simulink library "TURING_LOGIC"  (R2019b)
settings: Solver=VariableStepAuto  StartTime=0.0  StopTime=10.0  RelTol=1e-3
libraries: $bdroot x162, NOT x29, NAND x4
settings Model: Creator=jthur  LastModifiedBy=JTHURT

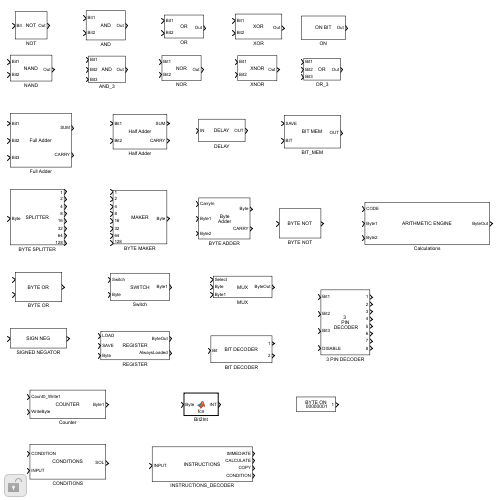
[thumbnail: Simulink's stored preview of the top-level diagram]
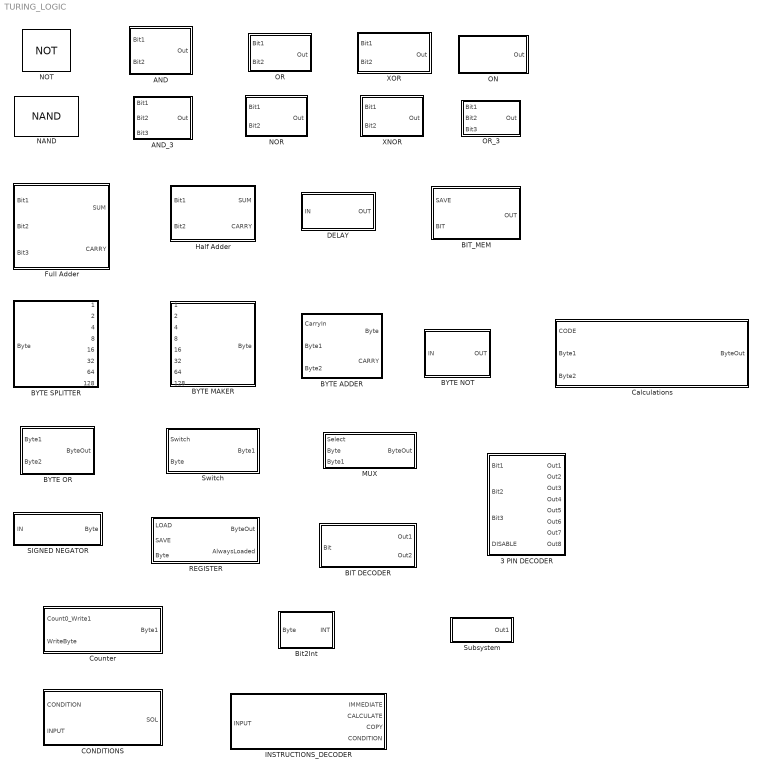
== system TURING_LOGIC ==
  3 PIN DECODER : Subsystem
      mask Display: fprintf("3 \n PIN \n DECODER")
  AND : Subsystem
      mask Display: fprintf("AND")
  AND_3 : Subsystem
      mask Display: fprintf("AND")
  BIT DECODER : Subsystem
      mask Display: fprintf("BIT DECODER")
  BIT_MEM : Subsystem
      mask Display: fprintf("BIT MEM")
  BYTE ADDER : Subsystem
      mask Display: fprintf("  Byte \n Adder")
  BYTE MAKER : Subsystem
      mask Display: fprintf("MAKER")
  BYTE NOT : Subsystem
      mask Display: fprintf("BYTE NOT")
  BYTE OR : Subsystem
      mask Display: fprintf("BYTE OR")
  "BYTE SPLITTER " : Subsystem
      mask Display: fprintf("SPLITTER")
  Bit2Int : MATLAB Function  TreatAsAtomicUnit=on
  CONDITIONS : Subsystem
      mask Display: fprintf("CONDITIONS")
  Calculations : Subsystem
      mask Display: fprintf("ARITHMETIC ENGINE")
  Counter : Subsystem
      mask Display: fprintf("COUNTER")
  DELAY : Subsystem
      mask Display: fprintf("DELAY")
  Full Adder : Subsystem
      mask Display: fprintf("Full Adder")
  Half Adder : Subsystem
      mask Display: fprintf("Half Adder")
  INSTRUCTIONS_DECODER : Subsystem
      mask Display: fprintf("INSTRUCTIONS")
  MUX : Subsystem
      mask Display: fprintf("MUX")
  NAND : NAND/NAND  SystemSampleTime=-1  Latency=0  AutoFrameSizeCalculation=off
  NOR : Subsystem
      mask Display: fprintf("NOR")
  NOT : NOT/NOT  SystemSampleTime=-1  Latency=0  AutoFrameSizeCalculation=off
  ON : Subsystem
      mask Display: fprintf("ON BIT")
  OR : Subsystem
      mask Display: fprintf("OR")
  OR_3 : Subsystem
      mask Display: fprintf("OR")
  REGISTER : Subsystem
      mask Display: fprintf("REGISTER")
  SIGNED NEGATOR : Subsystem
      mask Display: fprintf("SIGN NEG")
  Subsystem : Subsystem
      mask Display: fprintf("BYTE ON\n 00000001")
  Switch : Subsystem
      mask Display: fprintf("SWITCH")
  XNOR : Subsystem
      mask Display: fprintf("XNOR")
  XOR : Subsystem
      mask Display: fprintf("XOR")

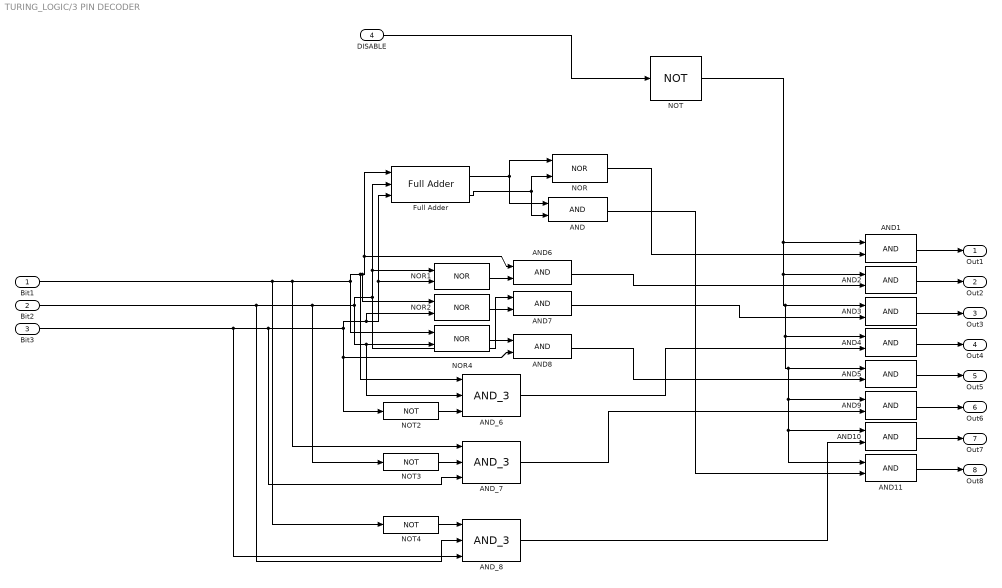
== system TURING_LOGIC/3 PIN DECODER ==
  Bit1 : Inport
  Bit2 : Inport  Port=2
  Bit3 : Inport  Port=3
  DISABLE : Inport  Port=4
  AND{,1..11} (12 alike) : $bdroot/AND  SystemSampleTime=-1  Latency=0  AutoFrameSizeCalculation=off
  AND_6 : $bdroot/AND_3  SystemSampleTime=-1  Latency=0  AutoFrameSizeCalculation=off
  AND_7 : $bdroot/AND_3  SystemSampleTime=-1  Latency=0  AutoFrameSizeCalculation=off
  AND_8 : $bdroot/AND_3  SystemSampleTime=-1  Latency=0  AutoFrameSizeCalculation=off
  Full Adder : $bdroot/Full Adder  SystemSampleTime=-1  Latency=0  AutoFrameSizeCalculation=off
  NOR{,1..2,4} (4 alike) : $bdroot/NOR  SystemSampleTime=-1  Latency=0  AutoFrameSizeCalculation=off
  NOT{,2..4} (4 alike) : NOT/NOT  SystemSampleTime=-1  Latency=0  AutoFrameSizeCalculation=off
  Out1 : Outport
  Out2 : Outport  Port=2
  Out3 : Outport  Port=3
  Out4 : Outport  Port=4
  Out5 : Outport  Port=5
  Out6 : Outport  Port=6
  Out7 : Outport  Port=7
  Out8 : Outport  Port=8
  wires:
  Bit3/1 -> AND_8/3, AND_7/3, NOR2/2, Full Adder/3, NOR1/2, NOT2/1, AND8/2
  Full Adder/2 -> NOR/2, AND/2
  Bit2/1 -> AND_8/2, NOT3/1, Full Adder/2, NOR1/1, AND7/1, AND_6/2, NOR4/2
  Bit1/1 -> NOT4/1, AND_7/1, AND_6/1, NOR2/1, Full Adder/1, AND6/1, NOR4/1
  NOT2/1 -> AND_6/3
  NOT3/1 -> AND_7/2
  NOR2/1 -> AND7/2
  NOR4/1 -> AND8/1
  NOR1/1 -> AND6/2
  NOT4/1 -> AND_8/1
  Full Adder/1 -> AND/1, NOR/1
  AND1/1 -> Out1/1
  AND2/1 -> Out2/1
  AND3/1 -> Out3/1
  AND4/1 -> Out4/1
  AND5/1 -> Out5/1
  AND9/1 -> Out6/1
  AND10/1 -> Out7/1
  AND11/1 -> Out8/1
  NOT/1 -> AND11/1, AND10/1, AND9/1, AND5/1, AND4/1, AND3/1, AND2/1, AND1/1
  AND/1 -> AND11/2
  NOR/1 -> AND1/2
  AND6/1 -> AND2/2
  AND7/1 -> AND3/2
  AND8/1 -> AND5/2
  AND_6/1 -> AND4/2
  AND_7/1 -> AND9/2
  AND_8/1 -> AND10/2
  DISABLE/1 -> NOT/1

== system TURING_LOGIC/AND ==
  Bit1 : Inport
  Bit2 : Inport  Port=2
  NAND1 : NAND/NAND  SystemSampleTime=-1  Latency=0  AutoFrameSizeCalculation=off
  NOT1 : NOT/NOT  SystemSampleTime=-1  Latency=0  AutoFrameSizeCalculation=off
  Out : Outport
  wires:
  NAND1/1 -> NOT1/1
  Bit1/1 -> NAND1/1
  NOT1/1 -> Out/1
  Bit2/1 -> NAND1/2

== system TURING_LOGIC/AND_3 ==
  Bit1 : Inport
  Bit2 : Inport  Port=2
  Bit3 : Inport  Port=3
  AND1 : $bdroot/AND  SystemSampleTime=-1  Latency=0  AutoFrameSizeCalculation=off
  AND2 : $bdroot/AND  SystemSampleTime=-1  Latency=0  AutoFrameSizeCalculation=off
  Out : Outport
  wires:
  AND1/1 -> AND2/1
  AND2/1 -> Out/1
  Bit1/1 -> AND1/1
  Bit3/1 -> AND2/2
  Bit2/1 -> AND1/2

== system TURING_LOGIC/BIT DECODER ==
  Bit : Inport
  AND : $bdroot/AND  SystemSampleTime=-1  Latency=0  AutoFrameSizeCalculation=off
  AND1 : $bdroot/AND  SystemSampleTime=-1  Latency=0  AutoFrameSizeCalculation=off
  NOT : NOT/NOT  SystemSampleTime=-1  Latency=0  AutoFrameSizeCalculation=off
  ON : $bdroot/ON  SystemSampleTime=-1  Latency=0  AutoFrameSizeCalculation=off
  Out1 : Outport
  Out2 : Outport  Port=2
  wires:
  ON/1 -> AND/2, AND1/2
  Bit/1 -> AND1/1, NOT/1
  NOT/1 -> AND/1
  AND/1 -> Out1/1
  AND1/1 -> Out2/1

== system TURING_LOGIC/BIT_MEM ==
  SAVE : Inport
  BIT : Inport  Port=2
  AND : $bdroot/AND  SystemSampleTime=-1  Latency=0  AutoFrameSizeCalculation=off
  AND1 : $bdroot/AND  SystemSampleTime=-1  Latency=0  AutoFrameSizeCalculation=off
  DELAY : $bdroot/DELAY  SystemSampleTime=-1  Latency=0  AutoFrameSizeCalculation=off
  NOR : $bdroot/NOR  SystemSampleTime=-1  Latency=0  AutoFrameSizeCalculation=off
  NOR1 : $bdroot/NOR  SystemSampleTime=-1  Latency=0  AutoFrameSizeCalculation=off
  NOT : NOT/NOT  SystemSampleTime=-1  Latency=0  AutoFrameSizeCalculation=off
  OUT : Outport
  wires:
  BIT/1 -> AND1/2, NOT/1
  NOT/1 -> AND/2
  SAVE/1 -> AND/1, AND1/1
  AND/1 -> NOR1/2
  NOR1/1 -> DELAY/1
  AND1/1 -> NOR/1
  NOR/1 -> NOR1/1
  DELAY/1 -> OUT/1, NOR/2

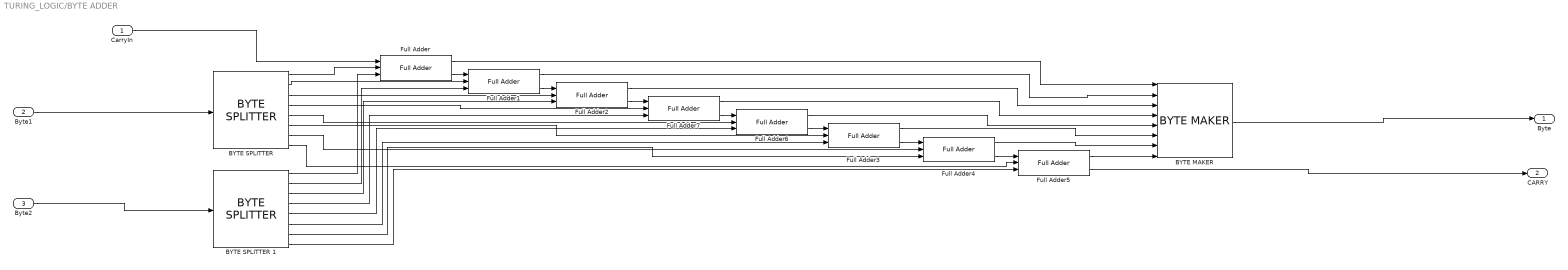
== system TURING_LOGIC/BYTE ADDER ==
  CarryIn : Inport
  Byte1 : Inport  Port=2
  Byte2 : Inport  Port=3
  BYTE MAKER : $bdroot/BYTE MAKER  SystemSampleTime=-1  Latency=0  AutoFrameSizeCalculation=off
  "BYTE SPLITTER " : $bdroot/BYTE SPLITTER   SystemSampleTime=-1  Latency=0  AutoFrameSizeCalculation=off
  BYTE SPLITTER 1 : $bdroot/BYTE SPLITTER   SystemSampleTime=-1  Latency=0  AutoFrameSizeCalculation=off
  Full Adder{,1..7} (8 alike) : $bdroot/Full Adder  SystemSampleTime=-1  Latency=0  AutoFrameSizeCalculation=off
  Byte : Outport
  CARRY : Outport  Port=2
  wires:
  BYTE SPLITTER 1/5 -> Full Adder6/3
  BYTE SPLITTER 1/3 -> Full Adder2/3
  "BYTE SPLITTER "/7 -> Full Adder4/2
  Full Adder1/1 -> BYTE MAKER/2
  BYTE SPLITTER 1/4 -> Full Adder7/3
  Full Adder3/2 -> Full Adder4/1
  "BYTE SPLITTER "/4 -> Full Adder7/2
  "BYTE SPLITTER "/5 -> Full Adder6/2
  Full Adder/1 -> BYTE MAKER/1
  Full Adder6/2 -> Full Adder3/1
  Full Adder3/1 -> BYTE MAKER/6
  Byte2/1 -> BYTE SPLITTER 1/1
  BYTE SPLITTER 1/6 -> Full Adder3/3
  BYTE SPLITTER 1/2 -> Full Adder1/3
  Full Adder/2 -> Full Adder1/1
  BYTE SPLITTER 1/8 -> Full Adder5/3
  Full Adder4/1 -> BYTE MAKER/7
  "BYTE SPLITTER "/2 -> Full Adder1/2
  Full Adder6/1 -> BYTE MAKER/5
  "BYTE SPLITTER "/1 -> Full Adder/2
  Full Adder2/1 -> BYTE MAKER/3
  Full Adder1/2 -> Full Adder2/1
  "BYTE SPLITTER "/3 -> Full Adder2/2
  Full Adder5/2 -> CARRY/1
  BYTE SPLITTER 1/1 -> Full Adder/3
  Full Adder7/1 -> BYTE MAKER/4
  "BYTE SPLITTER "/8 -> Full Adder5/2
  Full Adder5/1 -> BYTE MAKER/8
  "BYTE SPLITTER "/6 -> Full Adder3/2
  Full Adder2/2 -> Full Adder7/1
  BYTE SPLITTER 1/7 -> Full Adder4/3
  Full Adder7/2 -> Full Adder6/1
  CarryIn/1 -> Full Adder/1
  Full Adder4/2 -> Full Adder5/1
  BYTE MAKER/1 -> Byte/1
  Byte1/1 -> "BYTE SPLITTER "/1

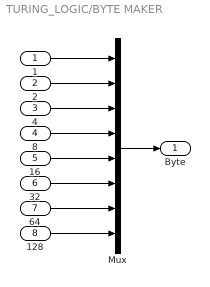
== system TURING_LOGIC/BYTE MAKER ==
  1 : Inport
  2 : Inport  Port=2
  4 : Inport  Port=3
  8 : Inport  Port=4
  16 : Inport  Port=5
  32 : Inport  Port=6
  64 : Inport  Port=7
  128 : Inport  Port=8
  Mux : Mux  Inputs=8
  Byte : Outport
  wires:
  1/1 -> Mux/1
  2/1 -> Mux/2
  4/1 -> Mux/3
  8/1 -> Mux/4
  16/1 -> Mux/5
  32/1 -> Mux/6
  64/1 -> Mux/7
  128/1 -> Mux/8
  Mux/1 -> Byte/1

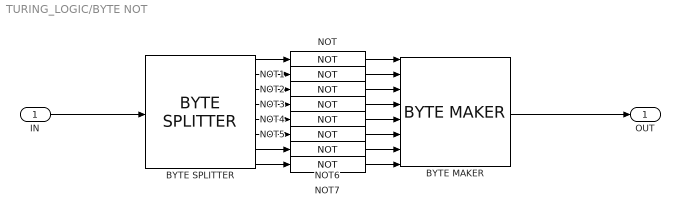
== system TURING_LOGIC/BYTE NOT ==
  IN : Inport
  BYTE MAKER : $bdroot/BYTE MAKER  SystemSampleTime=-1  Latency=0  AutoFrameSizeCalculation=off
  "BYTE SPLITTER " : $bdroot/BYTE SPLITTER   SystemSampleTime=-1  Latency=0  AutoFrameSizeCalculation=off
  NOT{,1..7} (8 alike) : NOT/NOT  SystemSampleTime=-1  Latency=0  AutoFrameSizeCalculation=off
  OUT : Outport
  wires:
  "BYTE SPLITTER "/8 -> NOT7/1
  NOT4/1 -> BYTE MAKER/5
  NOT/1 -> BYTE MAKER/1
  "BYTE SPLITTER "/3 -> NOT2/1
  "BYTE SPLITTER "/7 -> NOT6/1
  "BYTE SPLITTER "/4 -> NOT3/1
  NOT6/1 -> BYTE MAKER/7
  NOT7/1 -> BYTE MAKER/8
  "BYTE SPLITTER "/5 -> NOT4/1
  NOT2/1 -> BYTE MAKER/3
  NOT5/1 -> BYTE MAKER/6
  "BYTE SPLITTER "/2 -> NOT1/1
  NOT1/1 -> BYTE MAKER/2
  "BYTE SPLITTER "/1 -> NOT/1
  IN/1 -> "BYTE SPLITTER "/1
  NOT3/1 -> BYTE MAKER/4
  "BYTE SPLITTER "/6 -> NOT5/1
  BYTE MAKER/1 -> OUT/1

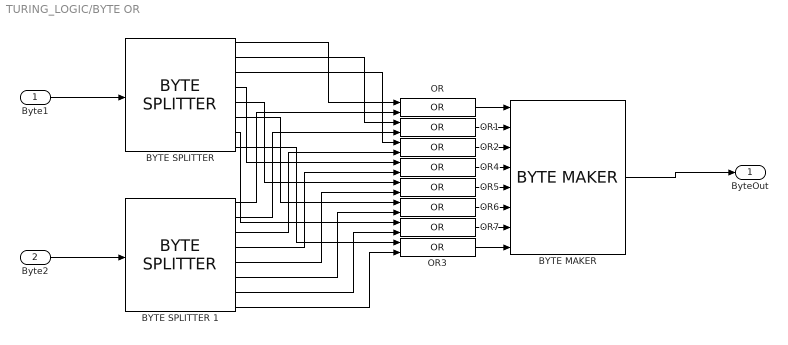
== system TURING_LOGIC/BYTE OR ==
  Byte1 : Inport
  Byte2 : Inport  Port=2
  BYTE MAKER : $bdroot/BYTE MAKER  SystemSampleTime=-1  Latency=0  AutoFrameSizeCalculation=off
  "BYTE SPLITTER " : $bdroot/BYTE SPLITTER   SystemSampleTime=-1  Latency=0  AutoFrameSizeCalculation=off
  BYTE SPLITTER 1 : $bdroot/BYTE SPLITTER   SystemSampleTime=-1  Latency=0  AutoFrameSizeCalculation=off
  OR{,1..7} (8 alike) : $bdroot/OR  SystemSampleTime=-1  Latency=0  AutoFrameSizeCalculation=off
  ByteOut : Outport
  wires:
  "BYTE SPLITTER "/2 -> OR1/1
  OR2/1 -> BYTE MAKER/3
  BYTE SPLITTER 1/2 -> OR1/2
  OR5/1 -> BYTE MAKER/5
  "BYTE SPLITTER "/3 -> OR2/1
  BYTE SPLITTER 1/1 -> OR/2
  BYTE SPLITTER 1/5 -> OR5/2
  BYTE SPLITTER 1/8 -> OR3/2
  BYTE SPLITTER 1/7 -> OR7/2
  "BYTE SPLITTER "/6 -> OR6/1
  OR3/1 -> BYTE MAKER/8
  BYTE SPLITTER 1/4 -> OR4/2
  BYTE SPLITTER 1/6 -> OR6/2
  BYTE SPLITTER 1/3 -> OR2/2
  Byte2/1 -> BYTE SPLITTER 1/1
  "BYTE SPLITTER "/4 -> OR4/1
  OR7/1 -> BYTE MAKER/7
  "BYTE SPLITTER "/5 -> OR5/1
  OR1/1 -> BYTE MAKER/2
  OR/1 -> BYTE MAKER/1
  OR4/1 -> BYTE MAKER/4
  "BYTE SPLITTER "/1 -> OR/1
  "BYTE SPLITTER "/8 -> OR3/1
  OR6/1 -> BYTE MAKER/6
  "BYTE SPLITTER "/7 -> OR7/1
  Byte1/1 -> "BYTE SPLITTER "/1
  BYTE MAKER/1 -> ByteOut/1

== system TURING_LOGIC/BYTE SPLITTER  ==
  Byte : Inport
  Demux : Demux  Outputs=8
  1 : Outport
  2 : Outport  Port=2
  4 : Outport  Port=3
  8 : Outport  Port=4
  16 : Outport  Port=5
  32 : Outport  Port=6
  64 : Outport  Port=7
  128 : Outport  Port=8
  wires:
  Byte/1 -> Demux/1
  Demux/1 -> 1/1
  Demux/2 -> 2/1
  Demux/3 -> 4/1
  Demux/4 -> 8/1
  Demux/5 -> 16/1
  Demux/6 -> 32/1
  Demux/7 -> 64/1
  Demux/8 -> 128/1

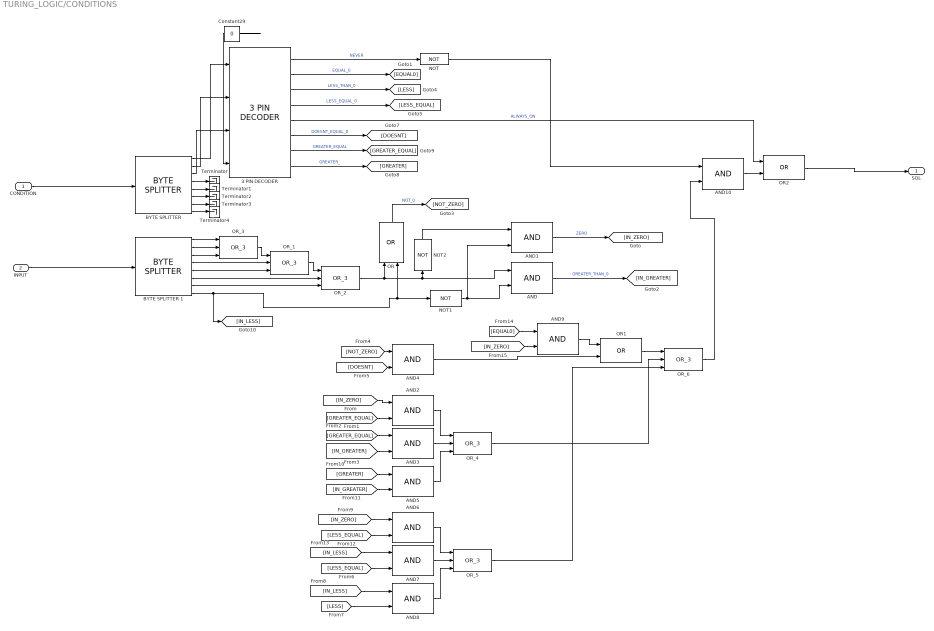
== system TURING_LOGIC/CONDITIONS ==
  CONDITION : Inport
  INPUT : Inport  Port=2
  3 PIN DECODER : $bdroot/3 PIN DECODER  SystemSampleTime=-1  Latency=0  AutoFrameSizeCalculation=off
  AND{,1..10} (11 alike) : $bdroot/AND  SystemSampleTime=-1  Latency=0  AutoFrameSizeCalculation=off
  "BYTE SPLITTER " : $bdroot/BYTE SPLITTER   SystemSampleTime=-1  Latency=0  AutoFrameSizeCalculation=off
  BYTE SPLITTER 1 : $bdroot/BYTE SPLITTER   SystemSampleTime=-1  Latency=0  AutoFrameSizeCalculation=off
  Constant29 : Constant  Value=0  SampleTime=-1
  NOT : NOT/NOT  SystemSampleTime=-1  Latency=0  AutoFrameSizeCalculation=off
  NOT1 : NOT/NOT  SystemSampleTime=-1  Latency=0  AutoFrameSizeCalculation=off
  NOT2 : NOT/NOT  SystemSampleTime=-1  Latency=0  AutoFrameSizeCalculation=off
  OR : $bdroot/OR  SystemSampleTime=-1  Latency=0  AutoFrameSizeCalculation=off
  OR1 : $bdroot/OR  SystemSampleTime=-1  Latency=0  AutoFrameSizeCalculation=off
  OR2 : $bdroot/OR  SystemSampleTime=-1  Latency=0  AutoFrameSizeCalculation=off
  OR_{1..6} (6 alike) : $bdroot/OR_3  SystemSampleTime=-1  Latency=0  AutoFrameSizeCalculation=off
  Terminator{,1..4} (5 alike) : Terminator
  SOL : Outport
  wires:
  [LESS_EQUAL] -> AND7/2
  BYTE SPLITTER 1/8 -> [IN_LESS], NOT1/1, OR/2
  BYTE SPLITTER 1/6 -> OR_2/2
  NOT1/1 -> AND1/2, AND/2
  [IN_ZERO] -> AND2/1
  BYTE SPLITTER 1/7 -> OR_2/3
  OR_6/1 -> AND10/2
  NOT2/1 -> AND1/1
  3 PIN DECODER/6 -> [DOESNT]  "DOESNT_EQUAL_0"
  OR_3/1 -> OR_1/1
  OR1/1 -> OR_6/1
  [IN_ZERO] -> AND6/1
  AND5/1 -> OR_4/3
  [IN_LESS] -> AND7/1
  "BYTE SPLITTER "/6 -> Terminator2/1
  [LESS] -> AND8/2
  OR_4/1 -> OR_6/2
  BYTE SPLITTER 1/3 -> OR_3/3
  [IN_LESS] -> AND8/1
  [EQUAL0] -> AND9/1
  [IN_GREATER] -> AND3/2
  3 PIN DECODER/7 -> [GREATER_EQUAL]  "GREATER_EQUAL"
  [IN_GREATER] -> AND5/2
  3 PIN DECODER/2 -> [EQUAL0]  "EQUAL_0"
  AND9/1 -> OR1/1
  OR_5/1 -> OR_6/3
  AND/1 -> [IN_GREATER]  "GREATER_THAN_0"
  AND10/1 -> OR2/2
  [DOESNT] -> AND4/2
  3 PIN DECODER/3 -> [LESS]  "LESS_THAN_0"
  "BYTE SPLITTER "/7 -> Terminator3/1
  3 PIN DECODER/5 -> OR2/1  "ALWAYS_ON"
  3 PIN DECODER/4 -> [LESS_EQUAL]  "LESS_EQUAL_0"
  "BYTE SPLITTER "/5 -> Terminator1/1
  BYTE SPLITTER 1/5 -> OR_1/3
  BYTE SPLITTER 1/2 -> OR_3/2
  AND6/1 -> OR_5/1
  "BYTE SPLITTER "/4 -> Terminator/1
  OR_2/1 -> OR/1, NOT2/1, AND/1
  AND1/1 -> [IN_ZERO]  "ZERO"
  [IN_ZERO] -> AND9/2
  AND7/1 -> OR_5/2
  AND2/1 -> OR_4/1
  [GREATER] -> AND5/1
  "BYTE SPLITTER "/8 -> Terminator4/1
  [GREATER_EQUAL] -> AND3/1
  [LESS_EQUAL] -> AND6/2
  OR_1/1 -> OR_2/1
  AND3/1 -> OR_4/2
  AND8/1 -> OR_5/3
  BYTE SPLITTER 1/4 -> OR_1/2
  NOT/1 -> AND10/1
  BYTE SPLITTER 1/1 -> OR_3/1
  OR/1 -> [NOT_ZERO]  "NOT_0"
  [NOT_ZERO] -> AND4/1
  3 PIN DECODER/1 -> NOT/1  "NEVER"
  [GREATER_EQUAL] -> AND2/2
  3 PIN DECODER/8 -> [GREATER]  "GREATER_"
  AND4/1 -> OR1/2
  CONDITION/1 -> "BYTE SPLITTER "/1
  OR2/1 -> SOL/1
  INPUT/1 -> BYTE SPLITTER 1/1
  "BYTE SPLITTER "/1 -> 3 PIN DECODER/1
  "BYTE SPLITTER "/2 -> 3 PIN DECODER/2
  "BYTE SPLITTER "/3 -> 3 PIN DECODER/3
  Constant29/1 -> 3 PIN DECODER/4

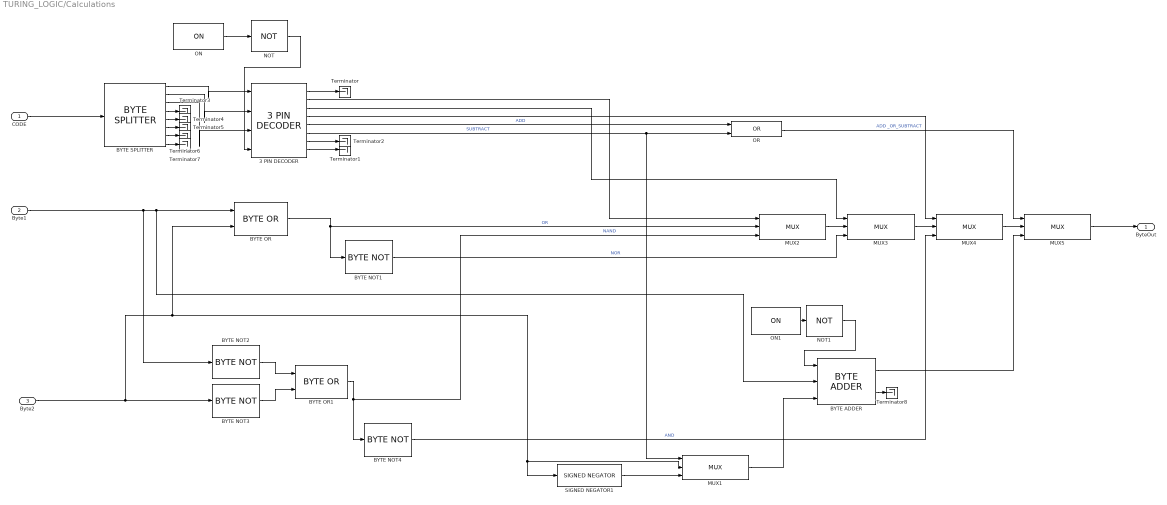
== system TURING_LOGIC/Calculations ==
  CODE : Inport
  Byte1 : Inport  Port=2
  Byte2 : Inport  Port=3
  3 PIN DECODER : $bdroot/3 PIN DECODER  SystemSampleTime=-1  Latency=0  AutoFrameSizeCalculation=off
  BYTE ADDER : $bdroot/BYTE ADDER  SystemSampleTime=-1  Latency=0  AutoFrameSizeCalculation=off
  BYTE NOT{1..4} (4 alike) : $bdroot/BYTE NOT  SystemSampleTime=-1  Latency=0  AutoFrameSizeCalculation=off
  BYTE OR : $bdroot/BYTE OR  SystemSampleTime=-1  Latency=0  AutoFrameSizeCalculation=off
  BYTE OR1 : $bdroot/BYTE OR  SystemSampleTime=-1  Latency=0  AutoFrameSizeCalculation=off
  "BYTE SPLITTER " : $bdroot/BYTE SPLITTER   SystemSampleTime=-1  Latency=0  AutoFrameSizeCalculation=off
  MUX{1..5} (5 alike) : $bdroot/MUX  SystemSampleTime=-1  Latency=0  AutoFrameSizeCalculation=off
  NOT : NOT/NOT  SystemSampleTime=-1  Latency=0  AutoFrameSizeCalculation=off
  NOT1 : NOT/NOT  SystemSampleTime=-1  Latency=0  AutoFrameSizeCalculation=off
  ON : $bdroot/ON  SystemSampleTime=-1  Latency=0  AutoFrameSizeCalculation=off
  ON1 : $bdroot/ON  SystemSampleTime=-1  Latency=0  AutoFrameSizeCalculation=off
  OR : $bdroot/OR  SystemSampleTime=-1  Latency=0  AutoFrameSizeCalculation=off
  SIGNED NEGATOR1 : $bdroot/SIGNED NEGATOR  SystemSampleTime=-1  Latency=0  AutoFrameSizeCalculation=off
  Terminator{,1..8} (9 alike) : Terminator
  ByteOut : Outport
  wires:
  OR/1 -> MUX5/1  "ADD _OR_SUBTRACT"
  3 PIN DECODER/6 -> OR/2, MUX1/1  "SUBTRACT"
  3 PIN DECODER/4 -> MUX4/1
  "BYTE SPLITTER "/6 -> Terminator5/1
  "BYTE SPLITTER "/2 -> 3 PIN DECODER/2
  BYTE NOT1/1 -> MUX3/3  "NOR"
  "BYTE SPLITTER "/5 -> Terminator4/1
  Byte1/1 -> BYTE NOT2/1, BYTE ADDER/2, BYTE OR/1
  3 PIN DECODER/7 -> Terminator2/1
  "BYTE SPLITTER "/7 -> Terminator6/1
  3 PIN DECODER/8 -> Terminator1/1
  3 PIN DECODER/1 -> Terminator/1
  BYTE ADDER/2 -> Terminator8/1
  NOT1/1 -> BYTE ADDER/1
  BYTE NOT2/1 -> BYTE OR1/1
  MUX3/1 -> MUX4/2
  "BYTE SPLITTER "/8 -> Terminator7/1
  MUX4/1 -> MUX5/2
  "BYTE SPLITTER "/3 -> 3 PIN DECODER/3
  Byte2/1 -> MUX1/2, SIGNED NEGATOR1/1, BYTE OR/2, BYTE NOT3/1
  "BYTE SPLITTER "/1 -> 3 PIN DECODER/1
  BYTE ADDER/1 -> MUX5/3
  ON/1 -> NOT/1
  3 PIN DECODER/5 -> OR/1  "ADD"
  BYTE OR1/1 -> MUX2/3, BYTE NOT4/1  "NAND"
  CODE/1 -> "BYTE SPLITTER "/1
  3 PIN DECODER/2 -> MUX2/1
  BYTE NOT3/1 -> BYTE OR1/2
  NOT/1 -> 3 PIN DECODER/4
  MUX1/1 -> BYTE ADDER/3
  BYTE OR/1 -> MUX2/2, BYTE NOT1/1  "OR"
  3 PIN DECODER/3 -> MUX3/1
  MUX2/1 -> MUX3/2
  BYTE NOT4/1 -> MUX4/3  "AND"
  SIGNED NEGATOR1/1 -> MUX1/3
  "BYTE SPLITTER "/4 -> Terminator3/1
  MUX5/1 -> ByteOut/1
  ON1/1 -> NOT1/1

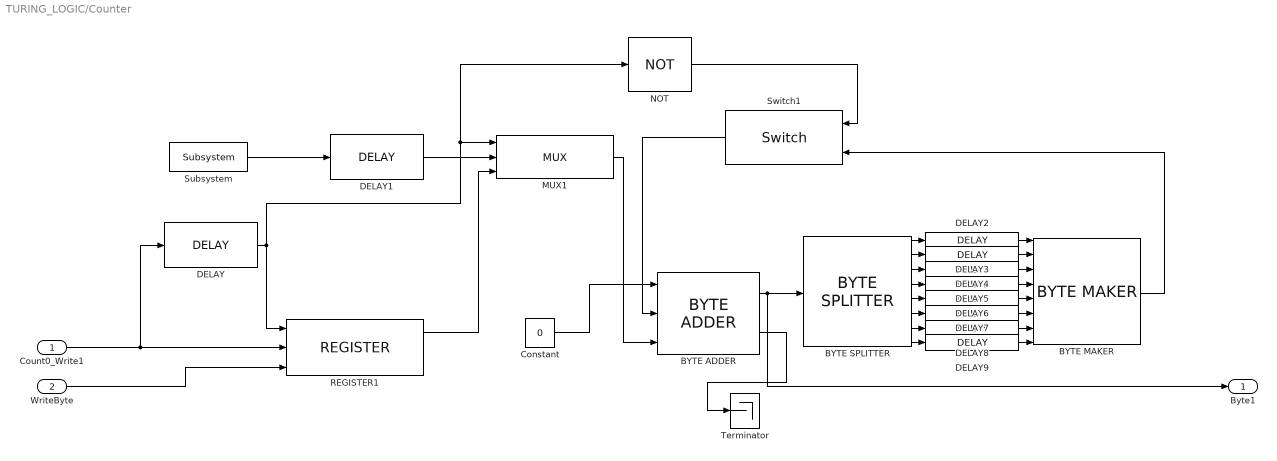
== system TURING_LOGIC/Counter ==
  Count0_Write1 : Inport
  WriteByte : Inport  Port=2
  BYTE ADDER : $bdroot/BYTE ADDER  SystemSampleTime=-1  Latency=0  AutoFrameSizeCalculation=off
  BYTE MAKER : $bdroot/BYTE MAKER  SystemSampleTime=-1  Latency=0  AutoFrameSizeCalculation=off
  "BYTE SPLITTER " : $bdroot/BYTE SPLITTER   SystemSampleTime=-1  Latency=0  AutoFrameSizeCalculation=off
  Constant : Constant  Value=0  SampleTime=-1
  DELAY{,1..9} (10 alike) : $bdroot/DELAY  SystemSampleTime=-1  Latency=0  AutoFrameSizeCalculation=off
  MUX1 : $bdroot/MUX  SystemSampleTime=-1  Latency=0  AutoFrameSizeCalculation=off
  NOT : NOT/NOT  SystemSampleTime=-1  Latency=0  AutoFrameSizeCalculation=off
  REGISTER1 : $bdroot/REGISTER  SystemSampleTime=-1  Latency=0  AutoFrameSizeCalculation=off
  Subsystem : $bdroot/Subsystem  SystemSampleTime=-1  Latency=0  AutoFrameSizeCalculation=off
  Switch1 : $bdroot/Switch  SystemSampleTime=-1  Latency=0  AutoFrameSizeCalculation=off
  Terminator : Terminator
  Byte1 : Outport
  wires:
  DELAY/1 -> NOT/1, MUX1/1, REGISTER1/1
  BYTE ADDER/1 -> "BYTE SPLITTER "/1, Byte1/1
  "BYTE SPLITTER "/3 -> DELAY4/1
  NOT/1 -> Switch1/1
  "BYTE SPLITTER "/8 -> DELAY9/1
  "BYTE SPLITTER "/7 -> DELAY8/1
  BYTE MAKER/1 -> Switch1/2
  Count0_Write1/1 -> DELAY/1, REGISTER1/2
  "BYTE SPLITTER "/5 -> DELAY6/1
  "BYTE SPLITTER "/2 -> DELAY3/1
  "BYTE SPLITTER "/4 -> DELAY5/1
  DELAY3/1 -> BYTE MAKER/2
  REGISTER1/1 -> MUX1/3
  DELAY1/1 -> MUX1/2
  "BYTE SPLITTER "/1 -> DELAY2/1
  Switch1/1 -> BYTE ADDER/2
  MUX1/1 -> BYTE ADDER/3
  "BYTE SPLITTER "/6 -> DELAY7/1
  DELAY2/1 -> BYTE MAKER/1
  DELAY8/1 -> BYTE MAKER/7
  DELAY6/1 -> BYTE MAKER/5
  DELAY7/1 -> BYTE MAKER/6
  DELAY4/1 -> BYTE MAKER/3
  DELAY5/1 -> BYTE MAKER/4
  DELAY9/1 -> BYTE MAKER/8
  WriteByte/1 -> REGISTER1/3
  Subsystem/1 -> DELAY1/1
  BYTE ADDER/2 -> Terminator/1
  Constant/1 -> BYTE ADDER/1

== system TURING_LOGIC/DELAY ==
  IN : Inport
  Unit Delay : UnitDelay  SampleTime=-1  HasFrameUpgradeWarning=on
  OUT : Outport
  wires:
  Unit Delay/1 -> OUT/1
  IN/1 -> Unit Delay/1

== system TURING_LOGIC/Full Adder ==
  Bit1 : Inport
  Bit2 : Inport  Port=2
  Bit3 : Inport  Port=3
  AND1 : $bdroot/AND  SystemSampleTime=-1  Latency=0  AutoFrameSizeCalculation=off
  AND2 : $bdroot/AND  SystemSampleTime=-1  Latency=0  AutoFrameSizeCalculation=off
  OR1 : $bdroot/OR  SystemSampleTime=-1  Latency=0  AutoFrameSizeCalculation=off
  XOR1 : $bdroot/XOR  SystemSampleTime=-1  Latency=0  AutoFrameSizeCalculation=off
  XOR2 : $bdroot/XOR  SystemSampleTime=-1  Latency=0  AutoFrameSizeCalculation=off
  SUM : Outport
  CARRY : Outport  Port=2
  wires:
  AND2/1 -> OR1/2
  XOR1/1 -> AND1/1, XOR2/1
  AND1/1 -> OR1/1
  OR1/1 -> CARRY/1  "CARRY"
  XOR2/1 -> SUM/1  "SUM"
  Bit1/1 -> AND2/1, XOR1/1
  Bit2/1 -> AND2/2, XOR1/2
  Bit3/1 -> XOR2/2, AND1/2

== system TURING_LOGIC/Half Adder ==
  Bit1 : Inport
  Bit2 : Inport  Port=2
  AND1 : $bdroot/AND  SystemSampleTime=-1  Latency=0  AutoFrameSizeCalculation=off
  XOR1 : $bdroot/XOR  SystemSampleTime=-1  Latency=0  AutoFrameSizeCalculation=off
  SUM : Outport
  CARRY : Outport  Port=2
  wires:
  Bit1/1 -> AND1/1, XOR1/1
  Bit2/1 -> AND1/2, XOR1/2
  AND1/1 -> CARRY/1  "CARRY"
  XOR1/1 -> SUM/1  "SUM"

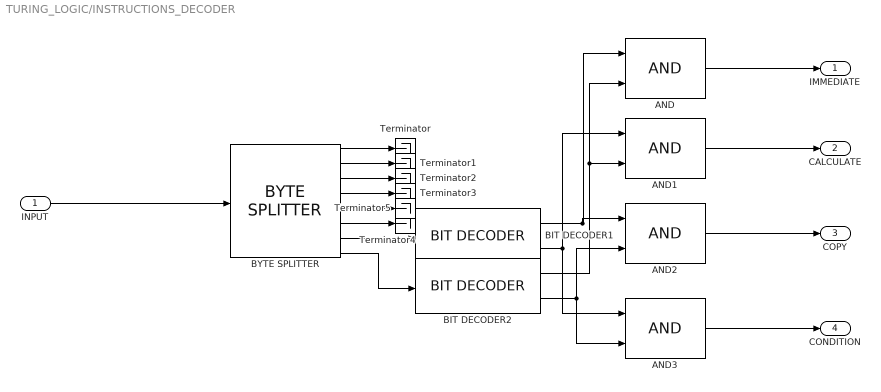
== system TURING_LOGIC/INSTRUCTIONS_DECODER ==
  INPUT : Inport
  AND{,1..3} (4 alike) : $bdroot/AND  SystemSampleTime=-1  Latency=0  AutoFrameSizeCalculation=off
  BIT DECODER1 : $bdroot/BIT DECODER  SystemSampleTime=-1  Latency=0  AutoFrameSizeCalculation=off
  BIT DECODER2 : $bdroot/BIT DECODER  SystemSampleTime=-1  Latency=0  AutoFrameSizeCalculation=off
  "BYTE SPLITTER " : $bdroot/BYTE SPLITTER   SystemSampleTime=-1  Latency=0  AutoFrameSizeCalculation=off
  Terminator{,1..5} (6 alike) : Terminator
  IMMEDIATE : Outport
  CALCULATE : Outport  Port=2
  COPY : Outport  Port=3
  CONDITION : Outport  Port=4
  wires:
  "BYTE SPLITTER "/8 -> BIT DECODER2/1
  "BYTE SPLITTER "/2 -> Terminator1/1
  "BYTE SPLITTER "/5 -> Terminator5/1
  "BYTE SPLITTER "/6 -> Terminator4/1
  BIT DECODER2/2 -> AND3/2, AND2/2
  "BYTE SPLITTER "/7 -> BIT DECODER1/1
  "BYTE SPLITTER "/3 -> Terminator2/1
  BIT DECODER1/2 -> AND1/1, AND3/1
  "BYTE SPLITTER "/1 -> Terminator/1
  BIT DECODER2/1 -> AND1/2, AND/2
  BIT DECODER1/1 -> AND2/1, AND/1
  INPUT/1 -> "BYTE SPLITTER "/1
  AND3/1 -> CONDITION/1
  "BYTE SPLITTER "/4 -> Terminator3/1
  AND/1 -> IMMEDIATE/1
  AND1/1 -> CALCULATE/1
  AND2/1 -> COPY/1

== system TURING_LOGIC/MUX ==
  Select : Inport
  Byte : Inport  Port=2
  Byte1 : Inport  Port=3
  BYTE OR : $bdroot/BYTE OR  SystemSampleTime=-1  Latency=0  AutoFrameSizeCalculation=off
  NOT : NOT/NOT  SystemSampleTime=-1  Latency=0  AutoFrameSizeCalculation=off
  Switch1 : $bdroot/Switch  SystemSampleTime=-1  Latency=0  AutoFrameSizeCalculation=off
  Switch2 : $bdroot/Switch  SystemSampleTime=-1  Latency=0  AutoFrameSizeCalculation=off
  ByteOut : Outport
  wires:
  Select/1 -> Switch2/1, NOT/1
  BYTE OR/1 -> ByteOut/1
  Switch1/1 -> BYTE OR/1
  Byte1/1 -> Switch2/2
  Switch2/1 -> BYTE OR/2
  NOT/1 -> Switch1/1
  Byte/1 -> Switch1/2

== system TURING_LOGIC/NOR ==
  Bit1 : Inport
  Bit2 : Inport  Port=2
  NOT : NOT/NOT  SystemSampleTime=-1  Latency=0  AutoFrameSizeCalculation=off
  OR : $bdroot/OR  SystemSampleTime=-1  Latency=0  AutoFrameSizeCalculation=off
  Out : Outport
  wires:
  Bit2/1 -> OR/2
  OR/1 -> NOT/1
  Bit1/1 -> OR/1
  NOT/1 -> Out/1

== system TURING_LOGIC/ON ==
  Constant : Constant
  NOT : NOT/NOT  SystemSampleTime=-1  Latency=0  AutoFrameSizeCalculation=off
  OR : $bdroot/OR  SystemSampleTime=-1  Latency=0  AutoFrameSizeCalculation=off
  Out : Outport
  wires:
  NOT/1 -> OR/2
  OR/1 -> Out/1
  Constant/1 -> NOT/1, OR/1

== system TURING_LOGIC/OR ==
  Bit1 : Inport
  Bit2 : Inport  Port=2
  NAND1 : NAND/NAND  SystemSampleTime=-1  Latency=0  AutoFrameSizeCalculation=off
  NOT1 : NOT/NOT  SystemSampleTime=-1  Latency=0  AutoFrameSizeCalculation=off
  NOT2 : NOT/NOT  SystemSampleTime=-1  Latency=0  AutoFrameSizeCalculation=off
  Out : Outport
  wires:
  Bit1/1 -> NOT1/1
  NOT1/1 -> NAND1/1
  NAND1/1 -> Out/1
  NOT2/1 -> NAND1/2
  Bit2/1 -> NOT2/1

== system TURING_LOGIC/OR_3 ==
  Bit1 : Inport
  Bit2 : Inport  Port=2
  Bit3 : Inport  Port=3
  OR1 : $bdroot/OR  SystemSampleTime=-1  Latency=0  AutoFrameSizeCalculation=off
  OR2 : $bdroot/OR  SystemSampleTime=-1  Latency=0  AutoFrameSizeCalculation=off
  Out : Outport
  wires:
  OR1/1 -> OR2/1
  Bit1/1 -> OR1/1
  Bit2/1 -> OR1/2
  Bit3/1 -> OR2/2
  OR2/1 -> Out/1

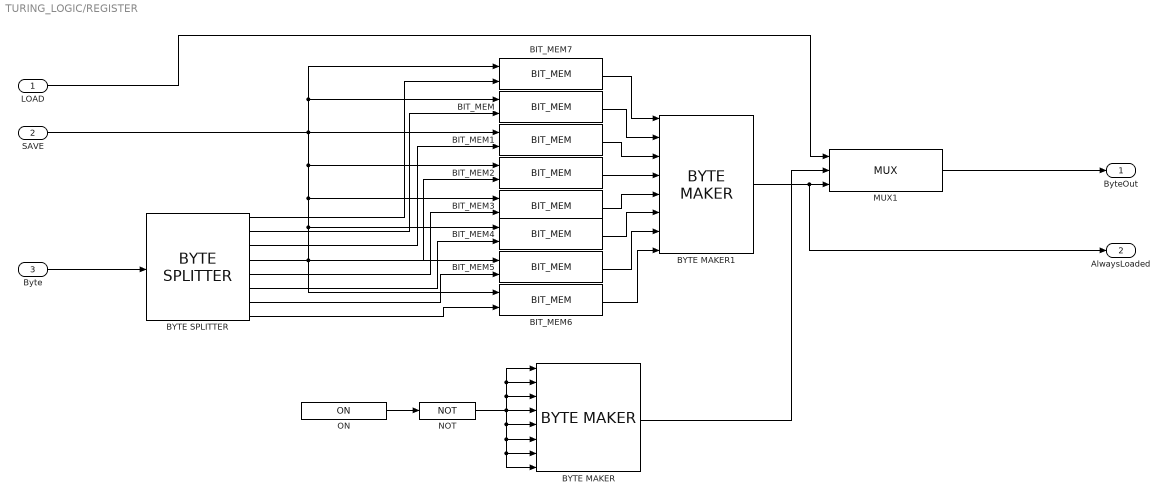
== system TURING_LOGIC/REGISTER ==
  LOAD : Inport
  SAVE : Inport  Port=2
  Byte : Inport  Port=3
  BIT_MEM{,1..7} (8 alike) : $bdroot/BIT_MEM  SystemSampleTime=-1  Latency=0  AutoFrameSizeCalculation=off
  BYTE MAKER : $bdroot/BYTE MAKER  SystemSampleTime=-1  Latency=0  AutoFrameSizeCalculation=off
  BYTE MAKER1 : $bdroot/BYTE MAKER  SystemSampleTime=-1  Latency=0  AutoFrameSizeCalculation=off
  "BYTE SPLITTER " : $bdroot/BYTE SPLITTER   SystemSampleTime=-1  Latency=0  AutoFrameSizeCalculation=off
  MUX1 : $bdroot/MUX  SystemSampleTime=-1  Latency=0  AutoFrameSizeCalculation=off
  NOT : NOT/NOT  SystemSampleTime=-1  Latency=0  AutoFrameSizeCalculation=off
  ON : $bdroot/ON  SystemSampleTime=-1  Latency=0  AutoFrameSizeCalculation=off
  ByteOut : Outport
  AlwaysLoaded : Outport  Port=2
  wires:
  "BYTE SPLITTER "/5 -> BIT_MEM3/2
  SAVE/1 -> BIT_MEM7/1, BIT_MEM/1, BIT_MEM2/1, BIT_MEM5/1, BIT_MEM6/1, BIT_MEM4/1, BIT_MEM3/1, BIT_MEM1/1
  BIT_MEM/1 -> BYTE MAKER1/2
  BIT_MEM5/1 -> BYTE MAKER1/7
  NOT/1 -> BYTE MAKER/5, BYTE MAKER/6, BYTE MAKER/8, BYTE MAKER/7, BYTE MAKER/2, BYTE MAKER/1, BYTE MAKER/3, BYTE MAKER/4
  BIT_MEM3/1 -> BYTE MAKER1/5
  "BYTE SPLITTER "/1 -> BIT_MEM7/2
  BIT_MEM4/1 -> BYTE MAKER1/6
  BIT_MEM2/1 -> BYTE MAKER1/4
  "BYTE SPLITTER "/7 -> BIT_MEM5/2
  "BYTE SPLITTER "/8 -> BIT_MEM6/2
  "BYTE SPLITTER "/3 -> BIT_MEM1/2
  MUX1/1 -> ByteOut/1
  BYTE MAKER1/1 -> AlwaysLoaded/1, MUX1/3
  "BYTE SPLITTER "/2 -> BIT_MEM/2
  "BYTE SPLITTER "/6 -> BIT_MEM4/2
  ON/1 -> NOT/1
  "BYTE SPLITTER "/4 -> BIT_MEM2/2
  BIT_MEM7/1 -> BYTE MAKER1/1
  BIT_MEM6/1 -> BYTE MAKER1/8
  BIT_MEM1/1 -> BYTE MAKER1/3
  BYTE MAKER/1 -> MUX1/2
  LOAD/1 -> MUX1/1
  Byte/1 -> "BYTE SPLITTER "/1

== system TURING_LOGIC/SIGNED NEGATOR ==
  IN : Inport
  BYTE ADDER : $bdroot/BYTE ADDER  SystemSampleTime=-1  Latency=0  AutoFrameSizeCalculation=off
  BYTE NOT1 : $bdroot/BYTE NOT  SystemSampleTime=-1  Latency=0  AutoFrameSizeCalculation=off
  Constant : Constant  Value=[0 0 0 0 0 0 0 0]  SampleTime=-1
  ON : $bdroot/ON  SystemSampleTime=-1  Latency=0  AutoFrameSizeCalculation=off
  Terminator : Terminator
  Byte : Outport
  wires:
  IN/1 -> BYTE NOT1/1
  BYTE NOT1/1 -> BYTE ADDER/2
  Constant/1 -> BYTE ADDER/3
  ON/1 -> BYTE ADDER/1
  BYTE ADDER/2 -> Terminator/1
  BYTE ADDER/1 -> Byte/1

== system TURING_LOGIC/Subsystem ==
  Constant : Constant  Value=[1 0 0 0 0 0 0 0]  SampleTime=-1
  Out1 : Outport
  wires:
  Constant/1 -> Out1/1

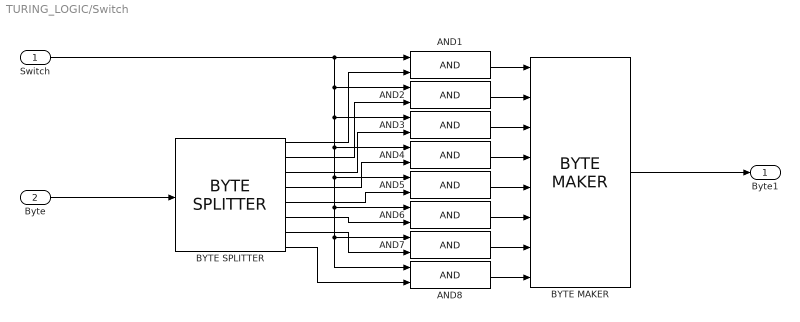
== system TURING_LOGIC/Switch ==
  Switch : Inport
  Byte : Inport  Port=2
  AND{1..8} (8 alike) : $bdroot/AND  SystemSampleTime=-1  Latency=0  AutoFrameSizeCalculation=off
  BYTE MAKER : $bdroot/BYTE MAKER  SystemSampleTime=-1  Latency=0  AutoFrameSizeCalculation=off
  "BYTE SPLITTER " : $bdroot/BYTE SPLITTER   SystemSampleTime=-1  Latency=0  AutoFrameSizeCalculation=off
  Byte1 : Outport
  wires:
  "BYTE SPLITTER "/6 -> AND6/2
  Switch/1 -> AND8/1, AND7/1, AND6/1, AND5/1, AND4/1, AND3/1, AND2/1, AND1/1
  AND2/1 -> BYTE MAKER/2
  AND3/1 -> BYTE MAKER/3
  AND4/1 -> BYTE MAKER/4
  "BYTE SPLITTER "/8 -> AND8/2
  Byte/1 -> "BYTE SPLITTER "/1
  "BYTE SPLITTER "/3 -> AND3/2
  "BYTE SPLITTER "/4 -> AND4/2
  "BYTE SPLITTER "/1 -> AND1/2
  AND7/1 -> BYTE MAKER/7
  "BYTE SPLITTER "/5 -> AND5/2
  "BYTE SPLITTER "/2 -> AND2/2
  "BYTE SPLITTER "/7 -> AND7/2
  AND6/1 -> BYTE MAKER/6
  AND1/1 -> BYTE MAKER/1
  AND5/1 -> BYTE MAKER/5
  AND8/1 -> BYTE MAKER/8
  BYTE MAKER/1 -> Byte1/1

== system TURING_LOGIC/XNOR ==
  Bit1 : Inport
  Bit2 : Inport  Port=2
  NOT : NOT/NOT  SystemSampleTime=-1  Latency=0  AutoFrameSizeCalculation=off
  XOR : $bdroot/XOR  SystemSampleTime=-1  Latency=0  AutoFrameSizeCalculation=off
  Out : Outport
  wires:
  NOT/1 -> Out/1
  XOR/1 -> NOT/1
  Bit1/1 -> XOR/1
  Bit2/1 -> XOR/2

== system TURING_LOGIC/XOR ==
  Bit1 : Inport
  Bit2 : Inport  Port=2
  AND : $bdroot/AND  SystemSampleTime=-1  Latency=0  AutoFrameSizeCalculation=off
  NAND : NAND/NAND  SystemSampleTime=-1  Latency=0  AutoFrameSizeCalculation=off
  OR : $bdroot/OR  SystemSampleTime=-1  Latency=0  AutoFrameSizeCalculation=off
  Out : Outport
  wires:
  Bit2/1 -> NAND/2, OR/2
  NAND/1 -> AND/1
  OR/1 -> AND/2
  AND/1 -> Out/1
  Bit1/1 -> NAND/1, OR/1

== matlab function TURING_LOGIC/Bit2Int ==
  data: Byte input; INT output
function INT = fcn(Byte)

BIT8 = [1 2 4 8 16 32 64 128];

INT = sum(Byte'.*BIT8);

end
